simulink model "ScriptDemo"  (R2022b)
settings: configuration reference "TmVcThermal_Configuration_sub" (kept outside this file)
undefined symbols (not defined in the file): aaaa, bbbb, cTmComprCtrl_D_u8HvacFlowTable_db, cTmComprCtrl_D_u8HvacFlowTable_sw, cTmComprCtrl_n_i16ChillCmpIMax, cTmComprCtrl_n_i16ChillCmpIMin, cTmComprCtrl_n_i16ChillCmpIMin666, cTmComprCtrl_n_i16ChillCmpPMax, cTmComprCtrl_n_i16ChillCmpPMin, cTmComprCtrl_n_i16CmpChillCoolRpmKiMax, cTmComprCtrl_n_i16CmpChillCoolRpmKiMin, cTmComprCtrl_n_i16CmpChillCoolRpmKpMax, cTmComprCtrl_n_i16CmpChillCoolRpmKpMin, cTmComprCtrl_n_i16CmpCoolRpmKiMax, cTmComprCtrl_n_i16CmpCoolRpmKiMin, cTmComprCtrl_n_i16CmpCoolRpmKpMax, cTmComprCtrl_n_i16CmpCoolRpmKpMin, cTmComprCtrl_n_i16SM4CmpHeatKiMax, cTmComprCtrl_n_i16SM4CmpHeatKiMin, cTmComprCtrl_n_i16SM4CmpHeatKpMax, cTmComprCtrl_n_i16SM4CmpHeatKpMin, cTmComprCtrl_n_i16SM5CmpHeatKiMax, cTmComprCtrl_n_i16SM5CmpHeatKiMin, cTmComprCtrl_n_i16SM5CmpHeatKpMax, cTmComprCtrl_n_i16SM5CmpHeatKpMin, cTmComprCtrl_n_i16SM6CmpHeatKiMax, cTmComprCtrl_n_i16SM6CmpHeatKiMin, cTmComprCtrl_n_i16SM6CmpHeatKpMax, cTmComprCtrl_n_i16SM6CmpHeatKpMin, cTmComprCtrl_n_u16CmpMaxSpdFanFltLimt, cTmComprCtrl_n_u16CmpMaxSpdLoSidePFltLimt, cTmComprCtrl_n_u16CmpMaxSpdSensorFltLimt, cTmComprCtrl_n_u16CompMinRpm, cTmComprCtrl_n_u16CompRpmIncThres, cTmComprCtrl_t_u16BattCooltFFPeriod, cTmComprCtrl_t_u16BattCooltPIPeriod, cTmComprCtrl_t_u16CmpCoolFFPeriod, cTmComprCtrl_t_u16CmpCoolPIPeriod, cTmComprCtrl_t_u16CoolCmpChillFFPeriod, cTmComprCtrl_t_u16CoolCmpChillPIPeriod, cTmComprCtrl_t_u16SM4CmpHeatFFPeriod, cTmComprCtrl_t_u16SM4CmpHeatPIPeriod, cTmComprCtrl_t_u16SM5CmpHeatFFPeriod, cTmComprCtrl_t_u16SM5CmpHeatPIPeriod, cTmComprCtrl_t_u16SM6CmpHeatFFPeriod, cTmComprCtrl_t_u16SM6CmpHeatPIPeriod, cTmComprCtrl_Te_EvapClearInteg, cTmComprCtrl_Te_i16HpReqTempSaturoffset, cTmComprCtrl_Te_i16SatLpReplaceDiff, cTmComprCtrl_Te_i16SM3BatDiffStartEvapDecOffset, cTmComprCtrl_Te_i16SM3EvapLo, cTmComprCtrl_Te_i16SM3TBatDiffEntEvapDecOffset, cTmComprCtrl_Te_i16SM3TBatDiffEntEvapDecOffsetQuit, cTmComprCtrl_Te_s32ErrCmpChillPIContinueCoolH, cTmComprCtrl_Te_s32ErrCmpChillPIContinueCoolL, cTmComprCtrl_Te_s32ErrCmpPIContinueChillH, cTmComprCtrl_Te_s32ErrCmpPIContinueChillL, cTmComprCtrl_Te_s32ErrCmpPIContinueCoolH, cTmComprCtrl_Te_s32ErrCmpPIContinueCoolL, cTmComprCtrl_Te_s32ErrCmpPIContinueHeatH ... (+398)
libraries: simulink x782, PCMULib x640, simulink_need_slupdate x4
(part 25 of 41)

== system ScriptDemo/Create/createMerge/After/SM3SM23/SM3SM1Error/NegAndPosCheck  ==
  SetPoint : Inport
  Acture : Inport  Port=2
  Compare To Constant : simulink/Logic and Bit Operations/Compare To Constant  relop=>=  const=0  OutDataTypeStr=boolean
  Data Type Conversion : DataTypeConversion  SaturateOnIntegerOverflow=off  RndMeth=Floor
  Data Type Conversion1 : DataTypeConversion  SaturateOnIntegerOverflow=off  RndMeth=Floor
  Data Type Conversion2 : DataTypeConversion  SaturateOnIntegerOverflow=off  RndMeth=Floor
  Sum : Sum  Inputs=|-+  OutDataTypeStr=Inherit: Same as first input
  Dvt : Outport  VectorParamsAs1DForOutWhenUnconnected=off
  Dvt_PosFlag : Outport  Port=2  VectorParamsAs1DForOutWhenUnconnected=off
  wires:
  SetPoint/1 -> Data Type Conversion/1
  Acture/1 -> Data Type Conversion1/1
  Sum/1 -> Data Type Conversion2/1
  Compare To Constant/1 -> Dvt_PosFlag/1
  Data Type Conversion/1 -> Sum/1
  Data Type Conversion1/1 -> Sum/2
  Data Type Conversion2/1 -> Compare To Constant/1, Dvt/1

== system ScriptDemo/Create/createMerge/After/SM3SM23/SM3SM2Error/NegAndPosCheck 1 ==
  SetPoint : Inport
  Acture : Inport  Port=2
  Compare To Constant : simulink/Logic and Bit Operations/Compare To Constant  relop=>=  const=0  OutDataTypeStr=boolean
  Data Type Conversion : DataTypeConversion  SaturateOnIntegerOverflow=off  RndMeth=Floor
  Data Type Conversion1 : DataTypeConversion  SaturateOnIntegerOverflow=off  RndMeth=Floor
  Data Type Conversion2 : DataTypeConversion  SaturateOnIntegerOverflow=off  RndMeth=Floor
  Sum : Sum  Inputs=|-+  OutDataTypeStr=Inherit: Same as first input
  Dvt : Outport  VectorParamsAs1DForOutWhenUnconnected=off
  Dvt_PosFlag : Outport  Port=2  VectorParamsAs1DForOutWhenUnconnected=off
  wires:
  Data Type Conversion2/1 -> Dvt/1, Compare To Constant/1
  Data Type Conversion1/1 -> Sum/2
  Data Type Conversion/1 -> Sum/1
  Compare To Constant/1 -> Dvt_PosFlag/1
  Sum/1 -> Data Type Conversion2/1
  Acture/1 -> Data Type Conversion1/1
  SetPoint/1 -> Data Type Conversion/1

== system ScriptDemo/Create/createMerge/After/SM3SM23/SM3_Ki/SM1Ki ==
  sTmSigProces_D_u8BattThermReq : Inport
  sTmIn_D_u8DCChrgSt : Inport  Port=2
  sTmSigProces_D_u8HvBattCoolgReq : Inport  Port=3
  Error : Inport  Port=4
  2-D Lookup Table10 : Lookup_n-D  LookupTableObject=mTmComprCtrl_n_u16FFBattCooltRpmCharging  BreakpointsForDimension1=mTmComprCtrl_n_u16KiBattCooltRpmSuperCharging_Y  BreakpointsForDimension2=mTmComprCtrl_n_u16KiBattCooltRpmSuperCharging_X  BreakpointsForDimension1DataTypeStr=Inherit: Inherit from 'Breakpoint data'  BreakpointsForDimension2DataTypeStr=Inherit: Inherit from 'Breakpoint data'  Table=mTmComprCtrl_n_u16KiBattCooltRpmSuperCharging  TableDataTypeStr=Inherit: Inherit from 'Table data'  ExtrapMethod=Clip  InternalRulePriority=Speed  OutDataTypeStr=Inherit: Inherit via back propagation  RndMeth=Simplest  InputSameDT=off
      settings: InputPortMap=u0,u1
  2-D Lookup Table8 : Lookup_n-D  LookupTableObject=mTmComprCtrl_n_u16FFBattCooltRpmCharging  BreakpointsForDimension1=mTmComprCtrl_n_u16KiBattCooltRpmNorm_Y  BreakpointsForDimension2=mTmComprCtrl_n_u16KiBattCooltRpmNorm_X  BreakpointsForDimension1DataTypeStr=Inherit: Inherit from 'Breakpoint data'  BreakpointsForDimension2DataTypeStr=Inherit: Inherit from 'Breakpoint data'  Table=mTmComprCtrl_n_u16KiBattCooltRpmNorm  TableDataTypeStr=Inherit: Inherit from 'Table data'  ExtrapMethod=Clip  InternalRulePriority=Speed  OutDataTypeStr=Inherit: Inherit via back propagation  RndMeth=Simplest  InputSameDT=off
      settings: InputPortMap=u0,u1
  2-D Lookup Table9 : Lookup_n-D  LookupTableObject=mTmComprCtrl_n_u16FFBattCooltRpmCharging  BreakpointsForDimension1=mTmComprCtrl_n_u16KiBattCooltRpmCharging_Y  BreakpointsForDimension2=mTmComprCtrl_n_u16KiBattCooltRpmCharging_X  BreakpointsForDimension1DataTypeStr=Inherit: Inherit from 'Breakpoint data'  BreakpointsForDimension2DataTypeStr=Inherit: Inherit from 'Breakpoint data'  Table=mTmComprCtrl_n_u16KiBattCooltRpmCharging  TableDataTypeStr=Inherit: Inherit from 'Table data'  ExtrapMethod=Clip  InternalRulePriority=Speed  OutDataTypeStr=Inherit: Inherit via back propagation  RndMeth=Simplest  InputSameDT=off
      settings: InputPortMap=u0,u1
  tableChoose : Subsystem
  SM1Ki : Outport
  wires:
  sTmIn_D_u8DCChrgSt/1 -> tableChoose/2(sTmIn_D_u8DCChrgSt)
  sTmSigProces_D_u8BattThermReq/1 -> tableChoose/1(sTmSigProces_D_u8BattThermReq)
  2-D Lookup Table10/1 -> tableChoose/5(tab3)
  2-D Lookup Table8/1 -> tableChoose/3(tab1)
  2-D Lookup Table9/1 -> tableChoose/4(tab2)
  tableChoose/1(out) -> SM1Ki/1
  sTmSigProces_D_u8HvBattCoolgReq/1 -> 2-D Lookup Table8/1, 2-D Lookup Table10/1, 2-D Lookup Table9/1
  Error/1 -> 2-D Lookup Table8/2, 2-D Lookup Table10/2, 2-D Lookup Table9/2

== system ScriptDemo/Create/createMerge/After/SM3SM23/SM3_Ki/SM2Ki ==
  Error : Inport
  sTmSigProces_Te_s32TAmb : Inport  Port=2  OutDataTypeStr=single
  sTmIn_X_s32ClimtRcirc : Inport  Port=3  OutDataTypeStr=single
  sTmComprCtrl_D_u8HvacFlowLevel : Inport  Port=4  OutDataTypeStr=uint8
  Flow2Rpm : Subsystem  mask{BlwHeatLevel_db=cTmComprCtrl_D_u8HvacFlowTable_db, BlwHeatLevel_sw=cTmComprCtrl_D_u8HvacFlowTable_sw, FFBlw1=mTmComprCtrl_n_u16KiCmpCoolRpm_RecFlow1, FFBlw1_Y=mTmComprCtrl_n_u16KiCmpCoolRpm_RecFlow1_Y, FFBlw1_X=mTmComprCtrl_n_u16KiCmpCoolRpm_RecFlow1_X, FFBlw3=mTmComprCtrl_n_u16KiCmpCoolRpm_RecFlow3, FFBlw3_Y=mTmComprCtrl_n_u16KiCmpCoolRpm_RecFlow3_Y, FFBlw3_X=mTmComprCtrl_n_u16KiCmpCoolRpm_RecFlow3_X, FFBlw5=mTmComprCtrl_n_u16KiCmpCoolRpm_RecFlow5, FFBlw5_Y=mTmComprCtrl_n_u16KiCmpCoolRpm_RecFlow5_Y, FFBlw5_X=mTmComprCtrl_n_u16KiCmpCoolRpm_RecFlow5_X, FFBlw7=mTmComprCtrl_n_u16KiCmpCoolRpm_RecFlow7, FFBlw7_Y=mTmComprCtrl_n_u16KiCmpCoolRpm_RecFlow7_Y, FFBlw7_X=mTmComprCtrl_n_u16KiCmpCoolRpm_RecFlow7_X, FFBlw9=mTmComprCtrl_n_u16KiCmpCoolRpm_RecFlow9, FFBlw9_Y=mTmComprCtrl_n_u16KiCmpCoolRpm_RecFlow9_Y, FFBlw9_X=mTmComprCtrl_n_u16KiCmpCoolRpm_RecFlow9_X}
      mask DialogControl ParameterGroupVar Prompt: 参数
  Flow2Rpm1 : Subsystem  mask{BlwHeatLevel_db=cTmComprCtrl_D_u8HvacFlowTable_db, BlwHeatLevel_sw=cTmComprCtrl_D_u8HvacFlowTable_sw, FFBlw1=mTmComprCtrl_n_u16KiCmpCoolRpm_OsaFlow1, FFBlw1_Y=mTmComprCtrl_n_u16KiCmpCoolRpm_OsaFlow1_Y, FFBlw1_X=mTmComprCtrl_n_u16KiCmpCoolRpm_OsaFlow1_X, FFBlw3=mTmComprCtrl_n_u16KiCmpCoolRpm_OsaFlow3, FFBlw3_Y=mTmComprCtrl_n_u16KiCmpCoolRpm_OsaFlow3_Y, FFBlw3_X=mTmComprCtrl_n_u16KiCmpCoolRpm_OsaFlow3_X, FFBlw5=mTmComprCtrl_n_u16KiCmpCoolRpm_OsaFlow5, FFBlw5_Y=mTmComprCtrl_n_u16KiCmpCoolRpm_OsaFlow5_Y, FFBlw5_X=mTmComprCtrl_n_u16KiCmpCoolRpm_OsaFlow5_X, FFBlw7=mTmComprCtrl_n_u16KiCmpCoolRpm_OsaFlow7, FFBlw7_Y=mTmComprCtrl_n_u16KiCmpCoolRpm_OsaFlow7_Y, FFBlw7_X=mTmComprCtrl_n_u16KiCmpCoolRpm_OsaFlow7_X, FFBlw9=mTmComprCtrl_n_u16KiCmpCoolRpm_OsaFlow9, FFBlw9_Y=mTmComprCtrl_n_u16KiCmpCoolRpm_OsaFlow9_Y, FFBlw9_X=mTmComprCtrl_n_u16KiCmpCoolRpm_OsaFlow9_X}
      mask DialogControl ParameterGroupVar Prompt: 参数
  interpolation : PCMULib/Calculation/interpolation  SystemSampleTime=-1  VariantActivationTime=update diagram  Latency=0  AutoFrameSizeCalculation=off
      settings: SourceProductName=PCMULib
  SM2Ki : Outport
  wires:
  Error/1 -> [Error]
  sTmSigProces_Te_s32TAmb/1 -> [sTmSigProces_Te_s32TAmb]
  sTmIn_X_s32ClimtRcirc/1 -> [sTmIn_X_s32ClimtRcirc]
  sTmComprCtrl_D_u8HvacFlowLevel/1 -> [sTmComprCtrl_D_u8HvacFlowLevel]
  Flow2Rpm/1(Flow2Rpm) -> interpolation/2  "mask"
  [sTmSigProces_Te_s32TAmb] -> Flow2Rpm/2(breakpoint1)
  [Error] -> Flow2Rpm/3(breakpoint2)
  [sTmComprCtrl_D_u8HvacFlowLevel] -> Flow2Rpm1/1(md_u8Blw)
  [sTmSigProces_Te_s32TAmb] -> Flow2Rpm1/2(breakpoint1)
  [sTmIn_X_s32ClimtRcirc] -> interpolation/1
  [sTmComprCtrl_D_u8HvacFlowLevel] -> Flow2Rpm/1(md_u8Blw)
  interpolation/1 -> SM2Ki/1
  Flow2Rpm1/1(Flow2Rpm) -> interpolation/3  "mask"
  [Error] -> Flow2Rpm1/3(breakpoint2)

== system ScriptDemo/Create/createMerge/After/SM3SM23/SM3_Ki/SM3SM1LikeKi ==
  sTmSigProces_D_u8BattThermReq : Inport
  sTmIn_D_u8DCChrgSt : Inport  Port=2
  sTmSigProces_D_u8HvBattCoolgReq : Inport  Port=3
  error : Inport  Port=4
  2-D Lookup Table5 : Lookup_n-D  LookupTableObject=mTmComprCtrl_n_u16FFBattCooltRpmCharging  BreakpointsForDimension1=mTmComprCtrl_n_u16KiSM3BattCooltRpmNorm_Y  BreakpointsForDimension2=mTmComprCtrl_n_u16KiSM3BattCooltRpmNorm_X  BreakpointsForDimension1DataTypeStr=Inherit: Inherit from 'Breakpoint data'  BreakpointsForDimension2DataTypeStr=Inherit: Inherit from 'Breakpoint data'  Table=mTmComprCtrl_n_u16KiSM3BattCooltRpmNorm  TableDataTypeStr=Inherit: Inherit from 'Table data'  ExtrapMethod=Clip  InternalRulePriority=Speed  OutDataTypeStr=Inherit: Inherit via back propagation  RndMeth=Simplest  InputSameDT=off
      settings: InputPortMap=u0,u1
  2-D Lookup Table6 : Lookup_n-D  LookupTableObject=mTmComprCtrl_n_u16FFBattCooltRpmCharging  BreakpointsForDimension1=mTmComprCtrl_n_u16KiSM3BattCooltRpmCharging_Y  BreakpointsForDimension2=mTmComprCtrl_n_u16KiSM3BattCooltRpmCharging_X  BreakpointsForDimension1DataTypeStr=Inherit: Inherit from 'Breakpoint data'  BreakpointsForDimension2DataTypeStr=Inherit: Inherit from 'Breakpoint data'  Table=mTmComprCtrl_n_u16KiSM3BattCooltRpmCharging  TableDataTypeStr=Inherit: Inherit from 'Table data'  ExtrapMethod=Clip  InternalRulePriority=Speed  OutDataTypeStr=Inherit: Inherit via back propagation  RndMeth=Simplest  InputSameDT=off
      settings: InputPortMap=u0,u1
  2-D Lookup Table7 : Lookup_n-D  LookupTableObject=mTmComprCtrl_n_u16FFBattCooltRpmCharging  BreakpointsForDimension1=mTmComprCtrl_n_u16KiSM3BattCooltRpmSuperCharging_Y  BreakpointsForDimension2=mTmComprCtrl_n_u16KiSM3BattCooltRpmSuperCharging_X  BreakpointsForDimension1DataTypeStr=Inherit: Inherit from 'Breakpoint data'  BreakpointsForDimension2DataTypeStr=Inherit: Inherit from 'Breakpoint data'  Table=mTmComprCtrl_n_u16KiSM3BattCooltRpmSuperCharging  TableDataTypeStr=Inherit: Inherit from 'Table data'  ExtrapMethod=Clip  InternalRulePriority=Speed  OutDataTypeStr=Inherit: Inherit via back propagation  RndMeth=Simplest  InputSameDT=off
      settings: InputPortMap=u0,u1
  tableChoose : Subsystem
  Ki : Outport  OutDataTypeStr=uint16
  wires:
  sTmIn_D_u8DCChrgSt/1 -> tableChoose/2(sTmIn_D_u8DCChrgSt)
  sTmSigProces_D_u8BattThermReq/1 -> tableChoose/1(sTmSigProces_D_u8BattThermReq)
  2-D Lookup Table7/1 -> tableChoose/5(tab3)
  2-D Lookup Table5/1 -> tableChoose/3(tab1)
  2-D Lookup Table6/1 -> tableChoose/4(tab2)
  sTmSigProces_D_u8HvBattCoolgReq/1 -> 2-D Lookup Table7/1, 2-D Lookup Table6/1, 2-D Lookup Table5/1
  error/1 -> 2-D Lookup Table7/2, 2-D Lookup Table6/2, 2-D Lookup Table5/2
  tableChoose/1(out) -> Ki/1

== system ScriptDemo/Create/createMerge/After/SM3SM23/SM3_Ki/SM3SM2LikeKi ==
  Error : Inport
  sTmSigProces_Te_s32TAmb : Inport  Port=2  OutDataTypeStr=single
  sTmIn_X_s32ClimtRcirc : Inport  Port=3  OutDataTypeStr=single
  sTmComprCtrl_D_u8HvacFlowLevel : Inport  Port=4  OutDataTypeStr=uint8
  Osa : Subsystem  mask{BlwHeatLevel_db=cTmComprCtrl_D_u8HvacFlowTable_db, BlwHeatLevel_sw=cTmComprCtrl_D_u8HvacFlowTable_sw, FFBlw1=mTmComprCtrl_n_u16KiSM3CmpCoolRpm_OsaFlow1, FFBlw1_Y=mTmComprCtrl_n_u16KiSM3CmpCoolRpm_OsaFlow1_Y, FFBlw1_X=mTmComprCtrl_n_u16KiSM3CmpCoolRpm_OsaFlow1_X, FFBlw3=mTmComprCtrl_n_u16KiSM3CmpCoolRpm_OsaFlow3, FFBlw3_Y=mTmComprCtrl_n_u16KiSM3CmpCoolRpm_OsaFlow3_Y, FFBlw3_X=mTmComprCtrl_n_u16KiSM3CmpCoolRpm_OsaFlow3_X, FFBlw5=mTmComprCtrl_n_u16KiSM3CmpCoolRpm_OsaFlow5, FFBlw5_Y=mTmComprCtrl_n_u16KiSM3CmpCoolRpm_OsaFlow5_Y, FFBlw5_X=mTmComprCtrl_n_u16KiSM3CmpCoolRpm_OsaFlow5_X, FFBlw7=mTmComprCtrl_n_u16KiSM3CmpCoolRpm_OsaFlow7, FFBlw7_Y=mTmComprCtrl_n_u16KiSM3CmpCoolRpm_OsaFlow7_Y, FFBlw7_X=mTmComprCtrl_n_u16KiSM3CmpCoolRpm_OsaFlow7_X, FFBlw9=mTmComprCtrl_n_u16KiSM3CmpCoolRpm_OsaFlow9, FFBlw9_Y=mTmComprCtrl_n_u16KiSM3CmpCoolRpm_OsaFlow9_Y, FFBlw9_X=mTmComprCtrl_n_u16KiSM3CmpCoolRpm_OsaFlow9_X}
      mask DialogControl ParameterGroupVar Prompt: 参数
  Rec : Subsystem  mask{BlwHeatLevel_db=cTmComprCtrl_D_u8HvacFlowTable_db, BlwHeatLevel_sw=cTmComprCtrl_D_u8HvacFlowTable_sw, FFBlw1=mTmComprCtrl_n_u16KiSM3CmpCoolRpm_RecFlow1, FFBlw1_Y=mTmComprCtrl_n_u16KiSM3CmpCoolRpm_RecFlow1_Y, FFBlw1_X=mTmComprCtrl_n_u16KiSM3CmpCoolRpm_RecFlow1_X, FFBlw3=mTmComprCtrl_n_u16KiSM3CmpCoolRpm_RecFlow3, FFBlw3_Y=mTmComprCtrl_n_u16KiSM3CmpCoolRpm_RecFlow3_Y, FFBlw3_X=mTmComprCtrl_n_u16KiSM3CmpCoolRpm_RecFlow3_X, FFBlw5=mTmComprCtrl_n_u16KiSM3CmpCoolRpm_RecFlow5, FFBlw5_Y=mTmComprCtrl_n_u16KiSM3CmpCoolRpm_RecFlow5_Y, FFBlw5_X=mTmComprCtrl_n_u16KiSM3CmpCoolRpm_RecFlow5_X, FFBlw7=mTmComprCtrl_n_u16KiSM3CmpCoolRpm_RecFlow7, FFBlw7_Y=mTmComprCtrl_n_u16KiSM3CmpCoolRpm_RecFlow7_Y, FFBlw7_X=mTmComprCtrl_n_u16KiSM3CmpCoolRpm_RecFlow7_X, FFBlw9=mTmComprCtrl_n_u16KiSM3CmpCoolRpm_RecFlow9, FFBlw9_Y=mTmComprCtrl_n_u16KiSM3CmpCoolRpm_RecFlow9_Y, FFBlw9_X=mTmComprCtrl_n_u16KiSM3CmpCoolRpm_RecFlow9_X}
      mask DialogControl ParameterGroupVar Prompt: 参数
  interpolation : PCMULib/Calculation/interpolation  SystemSampleTime=-1  VariantActivationTime=update diagram  Latency=0  AutoFrameSizeCalculation=off
      settings: SourceProductName=PCMULib
  Ki : Outport
  wires:
  interpolation/1 -> Ki/1
  [sTmIn_X_s32ClimtRcirc] -> interpolation/1
  Error/1 -> [Error]
  sTmSigProces_Te_s32TAmb/1 -> [sTmSigProces_Te_s32TAmb]
  sTmIn_X_s32ClimtRcirc/1 -> [sTmIn_X_s32ClimtRcirc]
  sTmComprCtrl_D_u8HvacFlowLevel/1 -> [sTmComprCtrl_D_u8HvacFlowLevel]
  [sTmComprCtrl_D_u8HvacFlowLevel] -> Rec/1(md_u8Blw)
  [sTmSigProces_Te_s32TAmb] -> Rec/2(breakpoint1)
  [Error] -> Rec/3(breakpoint2)
  [sTmComprCtrl_D_u8HvacFlowLevel] -> Osa/1(md_u8Blw)
  [sTmSigProces_Te_s32TAmb] -> Osa/2(breakpoint1)
  [Error] -> Osa/3(breakpoint2)
  Rec/1(Flow2Rpm) -> interpolation/2  "mask"
  Osa/1(Flow2Rpm) -> interpolation/3  "mask"

== system ScriptDemo/Create/createMerge/After/SM3SM23/SM3_Kp/SM1Kp ==
  sTmSigProces_D_u8BattThermReq : Inport
  sTmIn_D_u8DCChrgSt : Inport  Port=2
  sTmSigProces_D_u8HvBattCoolgReq : Inport  Port=3
  Error : Inport  Port=4
  2-D Lookup Table5 : Lookup_n-D  LookupTableObject=mTmComprCtrl_n_u16FFBattCooltRpmCharging  BreakpointsForDimension1=mTmComprCtrl_n_u16KpBattCooltRpmNorm_Y  BreakpointsForDimension2=mTmComprCtrl_n_u16KpBattCooltRpmNorm_X  BreakpointsForDimension1DataTypeStr=Inherit: Inherit from 'Breakpoint data'  BreakpointsForDimension2DataTypeStr=Inherit: Inherit from 'Breakpoint data'  Table=mTmComprCtrl_n_u16KpBattCooltRpmNorm  TableDataTypeStr=Inherit: Inherit from 'Table data'  ExtrapMethod=Clip  InternalRulePriority=Speed  OutDataTypeStr=Inherit: Inherit via back propagation  RndMeth=Simplest  InputSameDT=off
      settings: InputPortMap=u0,u1
  2-D Lookup Table6 : Lookup_n-D  LookupTableObject=mTmComprCtrl_n_u16FFBattCooltRpmCharging  BreakpointsForDimension1=mTmComprCtrl_n_u16KpBattCooltRpmCharging_Y  BreakpointsForDimension2=mTmComprCtrl_n_u16KpBattCooltRpmCharging_X  BreakpointsForDimension1DataTypeStr=Inherit: Inherit from 'Breakpoint data'  BreakpointsForDimension2DataTypeStr=Inherit: Inherit from 'Breakpoint data'  Table=mTmComprCtrl_n_u16KpBattCooltRpmCharging  TableDataTypeStr=Inherit: Inherit from 'Table data'  ExtrapMethod=Clip  InternalRulePriority=Speed  OutDataTypeStr=Inherit: Inherit via back propagation  RndMeth=Simplest  InputSameDT=off
      settings: InputPortMap=u0,u1
  2-D Lookup Table7 : Lookup_n-D  LookupTableObject=mTmComprCtrl_n_u16FFBattCooltRpmCharging  BreakpointsForDimension1=mTmComprCtrl_n_u16KpBattCooltRpmSuperCharging_Y  BreakpointsForDimension2=mTmComprCtrl_n_u16KpBattCooltRpmSuperCharging_X  BreakpointsForDimension1DataTypeStr=Inherit: Inherit from 'Breakpoint data'  BreakpointsForDimension2DataTypeStr=Inherit: Inherit from 'Breakpoint data'  Table=mTmComprCtrl_n_u16KpBattCooltRpmSuperCharging  TableDataTypeStr=Inherit: Inherit from 'Table data'  ExtrapMethod=Clip  InternalRulePriority=Speed  OutDataTypeStr=Inherit: Inherit via back propagation  RndMeth=Simplest  InputSameDT=off
      settings: InputPortMap=u0,u1
  tableChoose : Subsystem
  SM1Kp : Outport
  wires:
  sTmIn_D_u8DCChrgSt/1 -> tableChoose/2(sTmIn_D_u8DCChrgSt)
  sTmSigProces_D_u8BattThermReq/1 -> tableChoose/1(sTmSigProces_D_u8BattThermReq)
  2-D Lookup Table7/1 -> tableChoose/5(tab3)
  2-D Lookup Table5/1 -> tableChoose/3(tab1)
  2-D Lookup Table6/1 -> tableChoose/4(tab2)
  tableChoose/1(out) -> SM1Kp/1
  sTmSigProces_D_u8HvBattCoolgReq/1 -> 2-D Lookup Table7/1, 2-D Lookup Table6/1, 2-D Lookup Table5/1
  Error/1 -> 2-D Lookup Table7/2, 2-D Lookup Table6/2, 2-D Lookup Table5/2

== system ScriptDemo/Create/createMerge/After/SM3SM23/SM3_Kp/SM2Kp ==
  Error : Inport
  sTmSigProces_Te_s32TAmb : Inport  Port=2  OutDataTypeStr=single
  sTmIn_X_s32ClimtRcirc : Inport  Port=3  OutDataTypeStr=single
  sTmComprCtrl_D_u8HvacFlowLevel : Inport  Port=4  OutDataTypeStr=uint8
  Osa : Subsystem  mask{BlwHeatLevel_db=cTmComprCtrl_D_u8HvacFlowTable_db, BlwHeatLevel_sw=cTmComprCtrl_D_u8HvacFlowTable_sw, FFBlw1=mTmComprCtrl_n_u16KpCmpCoolRpm_OsaFlow1, FFBlw1_Y=mTmComprCtrl_n_u16KpCmpCoolRpm_OsaFlow1_Y, FFBlw1_X=mTmComprCtrl_n_u16KpCmpCoolRpm_OsaFlow1_X, FFBlw3=mTmComprCtrl_n_u16KpCmpCoolRpm_OsaFlow3, FFBlw3_Y=mTmComprCtrl_n_u16KpCmpCoolRpm_OsaFlow3_Y, FFBlw3_X=mTmComprCtrl_n_u16KpCmpCoolRpm_OsaFlow3_X, FFBlw5=mTmComprCtrl_n_u16KpCmpCoolRpm_OsaFlow5, FFBlw5_Y=mTmComprCtrl_n_u16KpCmpCoolRpm_OsaFlow5_Y, FFBlw5_X=mTmComprCtrl_n_u16KpCmpCoolRpm_OsaFlow5_X, FFBlw7=mTmComprCtrl_n_u16KpCmpCoolRpm_OsaFlow7, FFBlw7_Y=mTmComprCtrl_n_u16KpCmpCoolRpm_OsaFlow7_Y, FFBlw7_X=mTmComprCtrl_n_u16KpCmpCoolRpm_OsaFlow7_X, FFBlw9=mTmComprCtrl_n_u16KpCmpCoolRpm_OsaFlow9, FFBlw9_Y=mTmComprCtrl_n_u16KpCmpCoolRpm_OsaFlow9_Y, FFBlw9_X=mTmComprCtrl_n_u16KpCmpCoolRpm_OsaFlow9_X}
      mask DialogControl ParameterGroupVar Prompt: 参数
  Rec : Subsystem  mask{BlwHeatLevel_db=cTmComprCtrl_D_u8HvacFlowTable_db, BlwHeatLevel_sw=cTmComprCtrl_D_u8HvacFlowTable_sw, FFBlw1=mTmComprCtrl_n_u16KpCmpCoolRpm_RecFlow1, FFBlw1_Y=mTmComprCtrl_n_u16KpCmpCoolRpm_RecFlow1_Y, FFBlw1_X=mTmComprCtrl_n_u16KpCmpCoolRpm_RecFlow1_X, FFBlw3=mTmComprCtrl_n_u16KpCmpCoolRpm_RecFlow3, FFBlw3_Y=mTmComprCtrl_n_u16KpCmpCoolRpm_RecFlow3_Y, FFBlw3_X=mTmComprCtrl_n_u16KpCmpCoolRpm_RecFlow3_X, FFBlw5=mTmComprCtrl_n_u16KpCmpCoolRpm_RecFlow5, FFBlw5_Y=mTmComprCtrl_n_u16KpCmpCoolRpm_RecFlow5_Y, FFBlw5_X=mTmComprCtrl_n_u16KpCmpCoolRpm_RecFlow5_X, FFBlw7=mTmComprCtrl_n_u16KpCmpCoolRpm_RecFlow7, FFBlw7_Y=mTmComprCtrl_n_u16KpCmpCoolRpm_RecFlow7_Y, FFBlw7_X=mTmComprCtrl_n_u16KpCmpCoolRpm_RecFlow7_X, FFBlw9=mTmComprCtrl_n_u16KpCmpCoolRpm_RecFlow9, FFBlw9_Y=mTmComprCtrl_n_u16KpCmpCoolRpm_RecFlow9_Y, FFBlw9_X=mTmComprCtrl_n_u16KpCmpCoolRpm_RecFlow9_X}
      mask DialogControl ParameterGroupVar Prompt: 参数
  interpolation : PCMULib/Calculation/interpolation  SystemSampleTime=-1  VariantActivationTime=update diagram  Latency=0  AutoFrameSizeCalculation=off
      settings: SourceProductName=PCMULib
  SM2Kp : Outport
  wires:
  Error/1 -> [Error]
  sTmSigProces_Te_s32TAmb/1 -> [sTmSigProces_Te_s32TAmb]
  sTmIn_X_s32ClimtRcirc/1 -> [sTmIn_X_s32ClimtRcirc]
  sTmComprCtrl_D_u8HvacFlowLevel/1 -> [sTmComprCtrl_D_u8HvacFlowLevel]
  [Error] -> Rec/3(breakpoint2)
  [sTmSigProces_Te_s32TAmb] -> Rec/2(breakpoint1)
  Osa/1(Flow2Rpm) -> interpolation/3  "mask"
  [sTmIn_X_s32ClimtRcirc] -> interpolation/1
  [sTmComprCtrl_D_u8HvacFlowLevel] -> Rec/1(md_u8Blw)
  [Error] -> Osa/3(breakpoint2)
  [sTmSigProces_Te_s32TAmb] -> Osa/2(breakpoint1)
  Rec/1(Flow2Rpm) -> interpolation/2  "mask"
  [sTmComprCtrl_D_u8HvacFlowLevel] -> Osa/1(md_u8Blw)
  interpolation/1 -> SM2Kp/1

== system ScriptDemo/Create/createMerge/After/SM3SM23/SM3_Kp/SM3SM1LikeKp ==
  sTmSigProces_D_u8BattThermReq : Inport
  sTmIn_D_u8DCChrgSt : Inport  Port=2
  sTmSigProces_D_u8HvBattCoolgReq : Inport  Port=3
  error : Inport  Port=4
  2-D Lookup Table5 : Lookup_n-D  LookupTableObject=mTmComprCtrl_n_u16FFBattCooltRpmCharging  BreakpointsForDimension1=mTmComprCtrl_n_u16KpSM3BattCooltRpmNorm_Y  BreakpointsForDimension2=mTmComprCtrl_n_u16KpSM3BattCooltRpmNorm_X  BreakpointsForDimension1DataTypeStr=Inherit: Inherit from 'Breakpoint data'  BreakpointsForDimension2DataTypeStr=Inherit: Inherit from 'Breakpoint data'  Table=mTmComprCtrl_n_u16KpSM3BattCooltRpmNorm  TableDataTypeStr=Inherit: Inherit from 'Table data'  ExtrapMethod=Clip  InternalRulePriority=Speed  OutDataTypeStr=Inherit: Inherit via back propagation  RndMeth=Simplest  InputSameDT=off
      settings: InputPortMap=u0,u1
  2-D Lookup Table6 : Lookup_n-D  LookupTableObject=mTmComprCtrl_n_u16FFBattCooltRpmCharging  BreakpointsForDimension1=mTmComprCtrl_n_u16KpSM3BattCooltRpmCharging_Y  BreakpointsForDimension2=mTmComprCtrl_n_u16KpSM3BattCooltRpmCharging_X  BreakpointsForDimension1DataTypeStr=Inherit: Inherit from 'Breakpoint data'  BreakpointsForDimension2DataTypeStr=Inherit: Inherit from 'Breakpoint data'  Table=mTmComprCtrl_n_u16KpSM3BattCooltRpmCharging  TableDataTypeStr=Inherit: Inherit from 'Table data'  ExtrapMethod=Clip  InternalRulePriority=Speed  OutDataTypeStr=Inherit: Inherit via back propagation  RndMeth=Simplest  InputSameDT=off
      settings: InputPortMap=u0,u1
  2-D Lookup Table7 : Lookup_n-D  LookupTableObject=mTmComprCtrl_n_u16FFBattCooltRpmCharging  BreakpointsForDimension1=mTmComprCtrl_n_u16KpSM3BattCooltRpmSuperCharging_Y  BreakpointsForDimension2=mTmComprCtrl_n_u16KpSM3BattCooltRpmSuperCharging_X  BreakpointsForDimension1DataTypeStr=Inherit: Inherit from 'Breakpoint data'  BreakpointsForDimension2DataTypeStr=Inherit: Inherit from 'Breakpoint data'  Table=mTmComprCtrl_n_u16KpSM3BattCooltRpmSuperCharging  TableDataTypeStr=Inherit: Inherit from 'Table data'  ExtrapMethod=Clip  InternalRulePriority=Speed  OutDataTypeStr=Inherit: Inherit via back propagation  RndMeth=Simplest  InputSameDT=off
      settings: InputPortMap=u0,u1
  tableChoose : Subsystem
  Kp : Outport
  wires:
  sTmIn_D_u8DCChrgSt/1 -> tableChoose/2(sTmIn_D_u8DCChrgSt)
  sTmSigProces_D_u8BattThermReq/1 -> tableChoose/1(sTmSigProces_D_u8BattThermReq)
  2-D Lookup Table7/1 -> tableChoose/5(tab3)
  2-D Lookup Table5/1 -> tableChoose/3(tab1)
  2-D Lookup Table6/1 -> tableChoose/4(tab2)
  sTmSigProces_D_u8HvBattCoolgReq/1 -> 2-D Lookup Table7/1, 2-D Lookup Table6/1, 2-D Lookup Table5/1
  error/1 -> 2-D Lookup Table7/2, 2-D Lookup Table6/2, 2-D Lookup Table5/2
  tableChoose/1(out) -> Kp/1

== system ScriptDemo/Create/createMerge/After/SM3SM23/SM3_Kp/SM3SM2LikeKp ==
  Error : Inport
  sTmSigProces_Te_s32TAmb : Inport  Port=2  OutDataTypeStr=single
  sTmIn_X_s32ClimtRcirc : Inport  Port=3  OutDataTypeStr=single
  sTmComprCtrl_D_u8HvacFlowLevel : Inport  Port=4  OutDataTypeStr=uint8
  Osa : Subsystem  mask{BlwHeatLevel_db=cTmComprCtrl_D_u8HvacFlowTable_db, BlwHeatLevel_sw=cTmComprCtrl_D_u8HvacFlowTable_sw, FFBlw1=mTmComprCtrl_n_u16KpSM3CmpCoolRpm_OsaFlow1, FFBlw1_Y=mTmComprCtrl_n_u16KpSM3CmpCoolRpm_OsaFlow1_Y, FFBlw1_X=mTmComprCtrl_n_u16KpSM3CmpCoolRpm_OsaFlow1_X, FFBlw3=mTmComprCtrl_n_u16KpSM3CmpCoolRpm_OsaFlow3, FFBlw3_Y=mTmComprCtrl_n_u16KpSM3CmpCoolRpm_OsaFlow3_Y, FFBlw3_X=mTmComprCtrl_n_u16KpSM3CmpCoolRpm_OsaFlow3_X, FFBlw5=mTmComprCtrl_n_u16KpSM3CmpCoolRpm_OsaFlow5, FFBlw5_Y=mTmComprCtrl_n_u16KpSM3CmpCoolRpm_OsaFlow5_Y, FFBlw5_X=mTmComprCtrl_n_u16KpSM3CmpCoolRpm_OsaFlow5_X, FFBlw7=mTmComprCtrl_n_u16KpSM3CmpCoolRpm_OsaFlow7, FFBlw7_Y=mTmComprCtrl_n_u16KpSM3CmpCoolRpm_OsaFlow7_Y, FFBlw7_X=mTmComprCtrl_n_u16KpSM3CmpCoolRpm_OsaFlow7_X, FFBlw9=mTmComprCtrl_n_u16KpSM3CmpCoolRpm_OsaFlow9, FFBlw9_Y=mTmComprCtrl_n_u16KpSM3CmpCoolRpm_OsaFlow9_Y, FFBlw9_X=mTmComprCtrl_n_u16KpSM3CmpCoolRpm_OsaFlow9_X}
      mask DialogControl ParameterGroupVar Prompt: 参数
  Rec : Subsystem  mask{BlwHeatLevel_db=cTmComprCtrl_D_u8HvacFlowTable_db, BlwHeatLevel_sw=cTmComprCtrl_D_u8HvacFlowTable_sw, FFBlw1=mTmComprCtrl_n_u16KpSM3CmpCoolRpm_RecFlow1, FFBlw1_Y=mTmComprCtrl_n_u16KpSM3CmpCoolRpm_RecFlow1_Y, FFBlw1_X=mTmComprCtrl_n_u16KpSM3CmpCoolRpm_RecFlow1_X, FFBlw3=mTmComprCtrl_n_u16KpSM3CmpCoolRpm_RecFlow3, FFBlw3_Y=mTmComprCtrl_n_u16KpSM3CmpCoolRpm_RecFlow3_Y, FFBlw3_X=mTmComprCtrl_n_u16KpSM3CmpCoolRpm_RecFlow3_X, FFBlw5=mTmComprCtrl_n_u16KpSM3CmpCoolRpm_RecFlow5, FFBlw5_Y=mTmComprCtrl_n_u16KpSM3CmpCoolRpm_RecFlow5_Y, FFBlw5_X=mTmComprCtrl_n_u16KpSM3CmpCoolRpm_RecFlow5_X, FFBlw7=mTmComprCtrl_n_u16KpSM3CmpCoolRpm_RecFlow7, FFBlw7_Y=mTmComprCtrl_n_u16KpSM3CmpCoolRpm_RecFlow7_Y, FFBlw7_X=mTmComprCtrl_n_u16KpSM3CmpCoolRpm_RecFlow7_X, FFBlw9=mTmComprCtrl_n_u16KpSM3CmpCoolRpm_RecFlow9, FFBlw9_Y=mTmComprCtrl_n_u16KpSM3CmpCoolRpm_RecFlow9_Y, FFBlw9_X=mTmComprCtrl_n_u16KpSM3CmpCoolRpm_RecFlow9_X}
      mask DialogControl ParameterGroupVar Prompt: 参数
  interpolation : PCMULib/Calculation/interpolation  SystemSampleTime=-1  VariantActivationTime=update diagram  Latency=0  AutoFrameSizeCalculation=off
      settings: SourceProductName=PCMULib
  Kp : Outport
  wires:
  interpolation/1 -> Kp/1
  [sTmIn_X_s32ClimtRcirc] -> interpolation/1
  Error/1 -> [Error]
  sTmSigProces_Te_s32TAmb/1 -> [sTmSigProces_Te_s32TAmb]
  sTmIn_X_s32ClimtRcirc/1 -> [sTmIn_X_s32ClimtRcirc]
  sTmComprCtrl_D_u8HvacFlowLevel/1 -> [sTmComprCtrl_D_u8HvacFlowLevel]
  [sTmComprCtrl_D_u8HvacFlowLevel] -> Rec/1(md_u8Blw)
  [sTmSigProces_Te_s32TAmb] -> Rec/2(breakpoint1)
  [Error] -> Rec/3(breakpoint2)
  [sTmComprCtrl_D_u8HvacFlowLevel] -> Osa/1(md_u8Blw)
  [sTmSigProces_Te_s32TAmb] -> Osa/2(breakpoint1)
  [Error] -> Osa/3(breakpoint2)
  Rec/1(Flow2Rpm) -> interpolation/2  "mask"
  Osa/1(Flow2Rpm) -> interpolation/3  "mask"

== system ScriptDemo/Create/createMerge/After/SM4/ID26259_SM4Error/NegAndPosCheck 4 ==
  SetPoint : Inport
  Acture : Inport  Port=2
  Compare To Constant : simulink/Logic and Bit Operations/Compare To Constant  relop=>=  const=0  OutDataTypeStr=boolean
  Data Type Conversion : DataTypeConversion  SaturateOnIntegerOverflow=off  RndMeth=Floor
  Data Type Conversion1 : DataTypeConversion  SaturateOnIntegerOverflow=off  RndMeth=Floor
  Data Type Conversion2 : DataTypeConversion  SaturateOnIntegerOverflow=off  RndMeth=Floor
  Sum : Sum  Inputs=|-+  OutDataTypeStr=Inherit: Same as first input
  Dvt : Outport  VectorParamsAs1DForOutWhenUnconnected=off
  Dvt_PosFlag : Outport  Port=2  VectorParamsAs1DForOutWhenUnconnected=off
  wires:
  Data Type Conversion2/1 -> Dvt/1, Compare To Constant/1
  Data Type Conversion1/1 -> Sum/2
  Data Type Conversion/1 -> Sum/1
  Compare To Constant/1 -> Dvt_PosFlag/1
  Sum/1 -> Data Type Conversion2/1
  Acture/1 -> Data Type Conversion1/1
  SetPoint/1 -> Data Type Conversion/1

== system ScriptDemo/Create/createMerge/After/SM4/ID26259_SM4Error/NegAndPosCheck 5 ==
  SetPoint : Inport
  Acture : Inport  Port=2
  Compare To Constant : simulink/Logic and Bit Operations/Compare To Constant  relop=>=  const=0  OutDataTypeStr=boolean
  Data Type Conversion : DataTypeConversion  SaturateOnIntegerOverflow=off  RndMeth=Floor
  Data Type Conversion1 : DataTypeConversion  SaturateOnIntegerOverflow=off  RndMeth=Floor
  Data Type Conversion2 : DataTypeConversion  SaturateOnIntegerOverflow=off  RndMeth=Floor
  Sum : Sum  Inputs=|-+  OutDataTypeStr=Inherit: Same as first input
  Dvt : Outport  VectorParamsAs1DForOutWhenUnconnected=off
  Dvt_PosFlag : Outport  Port=2  VectorParamsAs1DForOutWhenUnconnected=off
  wires:
  Data Type Conversion2/1 -> Dvt/1, Compare To Constant/1
  Data Type Conversion1/1 -> Sum/2
  Data Type Conversion/1 -> Sum/1
  Compare To Constant/1 -> Dvt_PosFlag/1
  Sum/1 -> Data Type Conversion2/1
  Acture/1 -> Data Type Conversion1/1
  SetPoint/1 -> Data Type Conversion/1

== system ScriptDemo/Create/createMerge/After/SM4/ID26297_SM4FF/Flow2Rpm ==
  md_u8Blw : Inport
  breakpoint1 : Inport  Port=2
  breakpoint2 : Inport  Port=3
  2-D Lookup Table5 : Lookup_n-D  BreakpointsForDimension1=FFBlw1_Y  BreakpointsForDimension2=FFBlw1_X  BreakpointsForDimension1DataTypeStr=Inherit: Inherit from 'Breakpoint data'  BreakpointsForDimension2DataTypeStr=Inherit: Inherit from 'Breakpoint data'  Table=FFBlw1  TableDataTypeStr=Inherit: Inherit from 'Table data'  ExtrapMethod=Clip  InternalRulePriority=Speed  OutDataTypeStr=Inherit: Inherit from 'Table data'  RndMeth=Simplest
      settings: InputPortMap=u0,u1
  2-D Lookup Table6 : Lookup_n-D  BreakpointsForDimension1=FFBlw3_Y  BreakpointsForDimension2=FFBlw3_X  BreakpointsForDimension1DataTypeStr=Inherit: Inherit from 'Breakpoint data'  BreakpointsForDimension2DataTypeStr=Inherit: Inherit from 'Breakpoint data'  Table=FFBlw3  TableDataTypeStr=Inherit: Inherit from 'Table data'  ExtrapMethod=Clip  InternalRulePriority=Speed  OutDataTypeStr=Inherit: Inherit from 'Table data'  RndMeth=Simplest
      settings: InputPortMap=u0,u1
  2-D Lookup Table7 : Lookup_n-D  BreakpointsForDimension1=FFBlw5_Y  BreakpointsForDimension2=FFBlw5_X  BreakpointsForDimension1DataTypeStr=Inherit: Inherit from 'Breakpoint data'  BreakpointsForDimension2DataTypeStr=Inherit: Inherit from 'Breakpoint data'  Table=FFBlw5  TableDataTypeStr=Inherit: Inherit from 'Table data'  ExtrapMethod=Clip  InternalRulePriority=Speed  OutDataTypeStr=Inherit: Inherit from 'Table data'  RndMeth=Simplest
      settings: InputPortMap=u0,u1
  2-D Lookup Table8 : Lookup_n-D  BreakpointsForDimension1=FFBlw7_Y  BreakpointsForDimension2=FFBlw7_X  BreakpointsForDimension1DataTypeStr=Inherit: Inherit from 'Breakpoint data'  BreakpointsForDimension2DataTypeStr=Inherit: Inherit from 'Breakpoint data'  Table=FFBlw7  TableDataTypeStr=Inherit: Inherit from 'Table data'  ExtrapMethod=Clip  InternalRulePriority=Speed  OutDataTypeStr=Inherit: Inherit from 'Table data'  RndMeth=Simplest
      settings: InputPortMap=u0,u1
  2-D Lookup Table9 : Lookup_n-D  BreakpointsForDimension1=FFBlw9_Y  BreakpointsForDimension2=FFBlw9_X  BreakpointsForDimension1DataTypeStr=Inherit: Inherit from 'Breakpoint data'  BreakpointsForDimension2DataTypeStr=Inherit: Inherit from 'Breakpoint data'  Table=FFBlw9  TableDataTypeStr=Inherit: Inherit from 'Table data'  ExtrapMethod=Clip  InternalRulePriority=Speed  OutDataTypeStr=Inherit: Inherit from 'Table data'  RndMeth=Simplest
      settings: InputPortMap=u0,u1
  Add{2..6} (5 alike) : Sum  Inputs=+-  OutDataTypeStr=int16
  Add7 : Sum  Inputs=+++++  OutDataTypeStr=uint16
  Constant{,1..4} (5 alike) : Constant  Value=0.1  OutDataTypeStr=single
  Constant5 : Constant  Value=10  OutDataTypeStr=int16
  Constant6 : Constant  Value=20  OutDataTypeStr=int16
  Constant7 : Constant  Value=30  OutDataTypeStr=int16
  Constant8 : Constant  Value=40  OutDataTypeStr=int16
  Constant9 : Constant  Value=50  OutDataTypeStr=int16
  Data Type Conversion1 : DataTypeConversion  OutDataTypeStr=int16  SaturateOnIntegerOverflow=off  RndMeth=Floor
  Product{,1..9} (10 alike) : Product  OutDataTypeStr=single
  Subsystem1 : Subsystem
  Subsystem2 : Subsystem
  Subsystem3 : Subsystem
  Subsystem4 : Subsystem
  Subsystem5 : Subsystem
  XCP : Subsystem
  Flow2Rpm : Outport
  wires:
  Subsystem1/1(Out1) -> Product/2
  Product2/1 -> Product7/2
  [breakpoint2] -> 2-D Lookup Table5/2
  Product4/1 -> Product9/2
  Product9/1 -> Add7/5
  [breakpoint1] -> 2-D Lookup Table7/1
  Constant9/1 -> Add6/1
  [breakpoint1] -> 2-D Lookup Table9/1
  [breakpoint1] -> 2-D Lookup Table5/1
  [breakpoint1] -> 2-D Lookup Table6/1
  Product5/1 -> Add7/1
  2-D Lookup Table7/1 -> Product2/1
  Data Type Conversion1/1 -> Add4/2, Add6/2, Add5/2, Add3/2, Add2/2
  [breakpoint2] -> 2-D Lookup Table8/2
  Product/1 -> Product5/2
  Subsystem5/1(Out1) -> Product4/2
  [breakpoint2] -> 2-D Lookup Table7/2
  Subsystem2/1(Out1) -> Product1/2
  Constant8/1 -> Add5/1
  Product8/1 -> Add7/4
  Constant7/1 -> Add4/1
  Add4/1 -> Subsystem3/1(In1)
  Subsystem3/1(Out1) -> Product2/2
  Subsystem4/1(Out1) -> Product3/2
  Product1/1 -> Product6/2
  Add2/1 -> Subsystem1/1(In1)
  [breakpoint1] -> 2-D Lookup Table8/1
  [breakpoint2] -> 2-D Lookup Table6/2
  2-D Lookup Table5/1 -> Product/1
  Constant5/1 -> Add2/1
  2-D Lookup Table8/1 -> Product3/1
  Constant6/1 -> Add3/1
  Add6/1 -> Subsystem5/1(In1)
  Add5/1 -> Subsystem4/1(In1)
  Product3/1 -> Product8/2
  [breakpoint2] -> 2-D Lookup Table9/2
  Add3/1 -> Subsystem2/1(In1)
  Add7/1 -> Flow2Rpm/1
  2-D Lookup Table6/1 -> Product1/1
  Product7/1 -> Add7/3
  2-D Lookup Table9/1 -> Product4/1
  Product6/1 -> Add7/2
  breakpoint1/1 -> [breakpoint1]
  breakpoint2/1 -> [breakpoint2]
  XCP/1(Out1) -> Data Type Conversion1/1
  Constant/1 -> Product5/1
  Constant1/1 -> Product6/1
  Constant2/1 -> Product7/1
  Constant3/1 -> Product8/1
  Constant4/1 -> Product9/1
  md_u8Blw/1 -> XCP/1(md_u8Blw)

== system ScriptDemo/Create/createMerge/After/SM4/SM24FFEnable/PeriodTrig ==
  Counter_Reset : Inport
  Add : Sum
  Add1 : Sum  Inputs=+-
  Constant : Constant  Value=CounterLim
  Constant1 : Constant  Value=cTmSwArch_t_s32SampleTime
      settings: AttributesFormatString=%<Value>
  Constant2 : Constant  Value=0  OutDataTypeStr=single
  Constant50 : Constant  Value=cTmSwArch_t_s32SampleTime
      settings: AttributesFormatString=%<Value>
  Logical Operator : Logic  Operator=OR  AllPortsSameDT=off  OutDataTypeStr=boolean
  Relational Operator : RelationalOperator  OutDataTypeStr=boolean  RndMeth=Simplest  InputSameDT=off
  Switch : Switch  Criteria=u2 ~= 0  SaturateOnIntegerOverflow=off  InputSameDT=off
  Switch1 : Switch  Criteria=u2 ~= 0  SaturateOnIntegerOverflow=off  InputSameDT=off
  Unit Delay : UnitDelay  SampleTime=-1  HasFrameUpgradeWarning=on
  Unit Delay1 : UnitDelay  SampleTime=-1  HasFrameUpgradeWarning=on
  Counter_Trig : Outport
  wires:
  Relational Operator/1 -> Unit Delay1/1, Counter_Trig/1
  [CounterLim] -> Relational Operator/2
  Add/1 -> Unit Delay/1, Relational Operator/1
  Unit Delay/1 -> Switch/3
  Switch/1 -> Add/2
  Constant1/1 -> Add/1
  Logical Operator/1 -> Switch/2
  Counter_Reset/1 -> Switch1/2, Logical Operator/1
  Unit Delay1/1 -> Logical Operator/2
  Constant2/1 -> Switch1/3
  Switch1/1 -> Switch/1
  Add1/1 -> Switch1/1
  Constant50/1 -> Add1/2
  Constant/1 -> [CounterLim]
  [CounterLim] -> Add1/1

== system ScriptDemo/Create/createMerge/After/SM4/SM4_Ki/Flow2Rpm ==
  md_u8Blw : Inport
  breakpoint1 : Inport  Port=2
  breakpoint2 : Inport  Port=3
  2-D Lookup Table5 : Lookup_n-D  BreakpointsForDimension1=FFBlw1_Y  BreakpointsForDimension2=FFBlw1_X  BreakpointsForDimension1DataTypeStr=Inherit: Inherit from 'Breakpoint data'  BreakpointsForDimension2DataTypeStr=Inherit: Inherit from 'Breakpoint data'  Table=FFBlw1  TableDataTypeStr=Inherit: Inherit from 'Table data'  ExtrapMethod=Clip  InternalRulePriority=Speed  OutDataTypeStr=Inherit: Inherit from 'Table data'  RndMeth=Simplest
      settings: InputPortMap=u0,u1
  2-D Lookup Table6 : Lookup_n-D  BreakpointsForDimension1=FFBlw3_Y  BreakpointsForDimension2=FFBlw3_X  BreakpointsForDimension1DataTypeStr=Inherit: Inherit from 'Breakpoint data'  BreakpointsForDimension2DataTypeStr=Inherit: Inherit from 'Breakpoint data'  Table=FFBlw3  TableDataTypeStr=Inherit: Inherit from 'Table data'  ExtrapMethod=Clip  InternalRulePriority=Speed  OutDataTypeStr=Inherit: Inherit from 'Table data'  RndMeth=Simplest
      settings: InputPortMap=u0,u1
  2-D Lookup Table7 : Lookup_n-D  BreakpointsForDimension1=FFBlw5_Y  BreakpointsForDimension2=FFBlw5_X  BreakpointsForDimension1DataTypeStr=Inherit: Inherit from 'Breakpoint data'  BreakpointsForDimension2DataTypeStr=Inherit: Inherit from 'Breakpoint data'  Table=FFBlw5  TableDataTypeStr=Inherit: Inherit from 'Table data'  ExtrapMethod=Clip  InternalRulePriority=Speed  OutDataTypeStr=Inherit: Inherit from 'Table data'  RndMeth=Simplest
      settings: InputPortMap=u0,u1
  2-D Lookup Table8 : Lookup_n-D  BreakpointsForDimension1=FFBlw7_Y  BreakpointsForDimension2=FFBlw7_X  BreakpointsForDimension1DataTypeStr=Inherit: Inherit from 'Breakpoint data'  BreakpointsForDimension2DataTypeStr=Inherit: Inherit from 'Breakpoint data'  Table=FFBlw7  TableDataTypeStr=Inherit: Inherit from 'Table data'  ExtrapMethod=Clip  InternalRulePriority=Speed  OutDataTypeStr=Inherit: Inherit from 'Table data'  RndMeth=Simplest
      settings: InputPortMap=u0,u1
  2-D Lookup Table9 : Lookup_n-D  BreakpointsForDimension1=FFBlw9_Y  BreakpointsForDimension2=FFBlw9_X  BreakpointsForDimension1DataTypeStr=Inherit: Inherit from 'Breakpoint data'  BreakpointsForDimension2DataTypeStr=Inherit: Inherit from 'Breakpoint data'  Table=FFBlw9  TableDataTypeStr=Inherit: Inherit from 'Table data'  ExtrapMethod=Clip  InternalRulePriority=Speed  OutDataTypeStr=Inherit: Inherit from 'Table data'  RndMeth=Simplest
      settings: InputPortMap=u0,u1
  Add{2..6} (5 alike) : Sum  Inputs=+-  OutDataTypeStr=int16
  Add7 : Sum  Inputs=+++++  OutDataTypeStr=uint16
  Constant{,1..4} (5 alike) : Constant  Value=0.1  OutDataTypeStr=single
  Constant5 : Constant  Value=10  OutDataTypeStr=int16
  Constant6 : Constant  Value=20  OutDataTypeStr=int16
  Constant7 : Constant  Value=30  OutDataTypeStr=int16
  Constant8 : Constant  Value=40  OutDataTypeStr=int16
  Constant9 : Constant  Value=50  OutDataTypeStr=int16
  Data Type Conversion1 : DataTypeConversion  OutDataTypeStr=int16  SaturateOnIntegerOverflow=off  RndMeth=Floor
  Product{,1..9} (10 alike) : Product  OutDataTypeStr=single
  Subsystem1 : Subsystem
  Subsystem2 : Subsystem
  Subsystem3 : Subsystem
  Subsystem4 : Subsystem
  Subsystem5 : Subsystem
  XCP : Subsystem
  Flow2Rpm : Outport
  wires:
  Subsystem1/1(Out1) -> Product/2
  Product2/1 -> Product7/2
  [breakpoint2] -> 2-D Lookup Table5/2
  Product4/1 -> Product9/2
  Product9/1 -> Add7/5
  [breakpoint1] -> 2-D Lookup Table7/1
  Constant9/1 -> Add6/1
  [breakpoint1] -> 2-D Lookup Table9/1
  [breakpoint1] -> 2-D Lookup Table5/1
  [breakpoint1] -> 2-D Lookup Table6/1
  Product5/1 -> Add7/1
  2-D Lookup Table7/1 -> Product2/1
  Data Type Conversion1/1 -> Add4/2, Add6/2, Add5/2, Add3/2, Add2/2
  [breakpoint2] -> 2-D Lookup Table8/2
  Product/1 -> Product5/2
  Subsystem5/1(Out1) -> Product4/2
  [breakpoint2] -> 2-D Lookup Table7/2
  Subsystem2/1(Out1) -> Product1/2
  Constant8/1 -> Add5/1
  Product8/1 -> Add7/4
  Constant7/1 -> Add4/1
  Add4/1 -> Subsystem3/1(In1)
  Subsystem3/1(Out1) -> Product2/2
  Subsystem4/1(Out1) -> Product3/2
  Product1/1 -> Product6/2
  Add2/1 -> Subsystem1/1(In1)
  [breakpoint1] -> 2-D Lookup Table8/1
  [breakpoint2] -> 2-D Lookup Table6/2
  2-D Lookup Table5/1 -> Product/1
  Constant5/1 -> Add2/1
  2-D Lookup Table8/1 -> Product3/1
  Constant6/1 -> Add3/1
  Add6/1 -> Subsystem5/1(In1)
  Add5/1 -> Subsystem4/1(In1)
  Product3/1 -> Product8/2
  [breakpoint2] -> 2-D Lookup Table9/2
  Add3/1 -> Subsystem2/1(In1)
  Add7/1 -> Flow2Rpm/1
  2-D Lookup Table6/1 -> Product1/1
  Product7/1 -> Add7/3
  2-D Lookup Table9/1 -> Product4/1
  Product6/1 -> Add7/2
  breakpoint1/1 -> [breakpoint1]
  breakpoint2/1 -> [breakpoint2]
  XCP/1(Out1) -> Data Type Conversion1/1
  Constant/1 -> Product5/1
  Constant1/1 -> Product6/1
  Constant2/1 -> Product7/1
  Constant3/1 -> Product8/1
  Constant4/1 -> Product9/1
  md_u8Blw/1 -> XCP/1(md_u8Blw)

== system ScriptDemo/Create/createMerge/After/SM4/SM4_Kp/Flow2Rpm ==
  md_u8Blw : Inport
  breakpoint1 : Inport  Port=2
  breakpoint2 : Inport  Port=3
  2-D Lookup Table5 : Lookup_n-D  BreakpointsForDimension1=FFBlw1_Y  BreakpointsForDimension2=FFBlw1_X  BreakpointsForDimension1DataTypeStr=Inherit: Inherit from 'Breakpoint data'  BreakpointsForDimension2DataTypeStr=Inherit: Inherit from 'Breakpoint data'  Table=FFBlw1  TableDataTypeStr=Inherit: Inherit from 'Table data'  ExtrapMethod=Clip  InternalRulePriority=Speed  OutDataTypeStr=Inherit: Inherit from 'Table data'  RndMeth=Simplest
      settings: InputPortMap=u0,u1
  2-D Lookup Table6 : Lookup_n-D  BreakpointsForDimension1=FFBlw3_Y  BreakpointsForDimension2=FFBlw3_X  BreakpointsForDimension1DataTypeStr=Inherit: Inherit from 'Breakpoint data'  BreakpointsForDimension2DataTypeStr=Inherit: Inherit from 'Breakpoint data'  Table=FFBlw3  TableDataTypeStr=Inherit: Inherit from 'Table data'  ExtrapMethod=Clip  InternalRulePriority=Speed  OutDataTypeStr=Inherit: Inherit from 'Table data'  RndMeth=Simplest
      settings: InputPortMap=u0,u1
  2-D Lookup Table7 : Lookup_n-D  BreakpointsForDimension1=FFBlw5_Y  BreakpointsForDimension2=FFBlw5_X  BreakpointsForDimension1DataTypeStr=Inherit: Inherit from 'Breakpoint data'  BreakpointsForDimension2DataTypeStr=Inherit: Inherit from 'Breakpoint data'  Table=FFBlw5  TableDataTypeStr=Inherit: Inherit from 'Table data'  ExtrapMethod=Clip  InternalRulePriority=Speed  OutDataTypeStr=Inherit: Inherit from 'Table data'  RndMeth=Simplest
      settings: InputPortMap=u0,u1
  2-D Lookup Table8 : Lookup_n-D  BreakpointsForDimension1=FFBlw7_Y  BreakpointsForDimension2=FFBlw7_X  BreakpointsForDimension1DataTypeStr=Inherit: Inherit from 'Breakpoint data'  BreakpointsForDimension2DataTypeStr=Inherit: Inherit from 'Breakpoint data'  Table=FFBlw7  TableDataTypeStr=Inherit: Inherit from 'Table data'  ExtrapMethod=Clip  InternalRulePriority=Speed  OutDataTypeStr=Inherit: Inherit from 'Table data'  RndMeth=Simplest
      settings: InputPortMap=u0,u1
  2-D Lookup Table9 : Lookup_n-D  BreakpointsForDimension1=FFBlw9_Y  BreakpointsForDimension2=FFBlw9_X  BreakpointsForDimension1DataTypeStr=Inherit: Inherit from 'Breakpoint data'  BreakpointsForDimension2DataTypeStr=Inherit: Inherit from 'Breakpoint data'  Table=FFBlw9  TableDataTypeStr=Inherit: Inherit from 'Table data'  ExtrapMethod=Clip  InternalRulePriority=Speed  OutDataTypeStr=Inherit: Inherit from 'Table data'  RndMeth=Simplest
      settings: InputPortMap=u0,u1
  Add{2..6} (5 alike) : Sum  Inputs=+-  OutDataTypeStr=int16
  Add7 : Sum  Inputs=+++++  OutDataTypeStr=uint16
  Constant{,1..4} (5 alike) : Constant  Value=0.1  OutDataTypeStr=single
  Constant5 : Constant  Value=10  OutDataTypeStr=int16
  Constant6 : Constant  Value=20  OutDataTypeStr=int16
  Constant7 : Constant  Value=30  OutDataTypeStr=int16
  Constant8 : Constant  Value=40  OutDataTypeStr=int16
  Constant9 : Constant  Value=50  OutDataTypeStr=int16
  Data Type Conversion1 : DataTypeConversion  OutDataTypeStr=int16  SaturateOnIntegerOverflow=off  RndMeth=Floor
  Product{,1..9} (10 alike) : Product  OutDataTypeStr=single
  Subsystem1 : Subsystem
  Subsystem2 : Subsystem
  Subsystem3 : Subsystem
  Subsystem4 : Subsystem
  Subsystem5 : Subsystem
  XCP : Subsystem
  Flow2Rpm : Outport
  wires:
  Subsystem1/1(Out1) -> Product/2
  Product2/1 -> Product7/2
  [breakpoint2] -> 2-D Lookup Table5/2
  Product4/1 -> Product9/2
  Product9/1 -> Add7/5
  [breakpoint1] -> 2-D Lookup Table7/1
  Constant9/1 -> Add6/1
  [breakpoint1] -> 2-D Lookup Table9/1
  [breakpoint1] -> 2-D Lookup Table5/1
  [breakpoint1] -> 2-D Lookup Table6/1
  Product5/1 -> Add7/1
  2-D Lookup Table7/1 -> Product2/1
  Data Type Conversion1/1 -> Add4/2, Add6/2, Add5/2, Add3/2, Add2/2
  [breakpoint2] -> 2-D Lookup Table8/2
  Product/1 -> Product5/2
  Subsystem5/1(Out1) -> Product4/2
  [breakpoint2] -> 2-D Lookup Table7/2
  Subsystem2/1(Out1) -> Product1/2
  Constant8/1 -> Add5/1
  Product8/1 -> Add7/4
  Constant7/1 -> Add4/1
  Add4/1 -> Subsystem3/1(In1)
  Subsystem3/1(Out1) -> Product2/2
  Subsystem4/1(Out1) -> Product3/2
  Product1/1 -> Product6/2
  Add2/1 -> Subsystem1/1(In1)
  [breakpoint1] -> 2-D Lookup Table8/1
  [breakpoint2] -> 2-D Lookup Table6/2
  2-D Lookup Table5/1 -> Product/1
  Constant5/1 -> Add2/1
  2-D Lookup Table8/1 -> Product3/1
  Constant6/1 -> Add3/1
  Add6/1 -> Subsystem5/1(In1)
  Add5/1 -> Subsystem4/1(In1)
  Product3/1 -> Product8/2
  [breakpoint2] -> 2-D Lookup Table9/2
  Add3/1 -> Subsystem2/1(In1)
  Add7/1 -> Flow2Rpm/1
  2-D Lookup Table6/1 -> Product1/1
  Product7/1 -> Add7/3
  2-D Lookup Table9/1 -> Product4/1
  Product6/1 -> Add7/2
  breakpoint1/1 -> [breakpoint1]
  breakpoint2/1 -> [breakpoint2]
  XCP/1(Out1) -> Data Type Conversion1/1
  Constant/1 -> Product5/1
  Constant1/1 -> Product6/1
  Constant2/1 -> Product7/1
  Constant3/1 -> Product8/1
  Constant4/1 -> Product9/1
  md_u8Blw/1 -> XCP/1(md_u8Blw)
